simulink model "AIL_STATE_MACHINE"  (R2021b)
settings: Solver=FixedStepDiscrete  StartTime=0.0  StopTime=20  FixedStep=1e-3  RelTol=1e-3
undefined symbols (not defined in the file): BUCU3_FCC1_LHACTCMDVSCURRENTVALID, BUCU3_FCC1_LHACTCTLVSMONLOOPVALID, BUCU3_FCC1_LHACTPOSVSCMDVALID, BUCU3_FCC1_LHELEVPOSITIONVALID, BUCU3_FCC1_LHGEARINGVALID, BUCU3_FCC1_LHHYDPRESSVALID, BUCU3_FCC1_LHPOWERVALID, BUCU3_FCC1_LHSPEEDINPUTVALID, sigbuilder_block
libraries: simulink x5, LATCH_ERROR_LIB x1
settings Model: Creator=C83127  LastModifiedBy=ACH

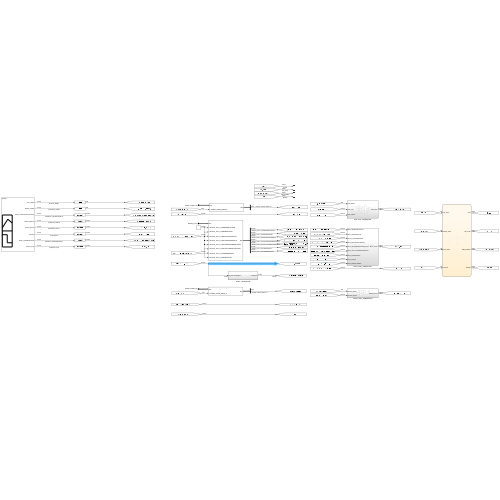
[thumbnail: Simulink's stored preview of the top-level diagram]
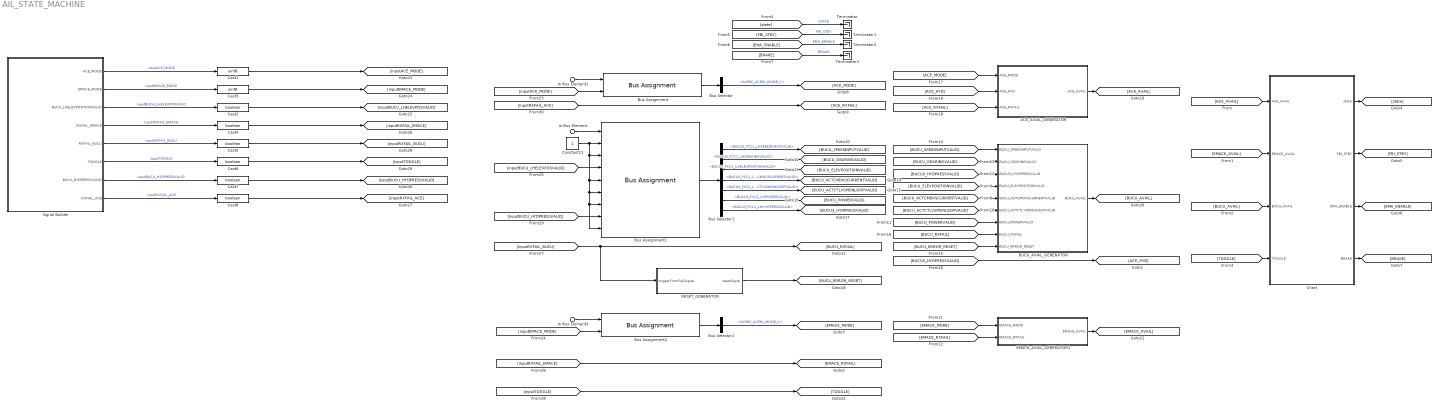
== system AIL_STATE_MACHINE ==
  In Bus Element : Inport  PortName=BUCU3_FCC1
  In Bus Element1 : Inport  Port=2  PortName=ACE9C_ACE8x_9C
  In Bus Element3 : Inport  Port=3  PortName=ACE8C_ACE9x_8C
  ACE_AVAIL_GENERATOR : Subsystem
  BUCU_AVAIL_GENERATOR : Subsystem
  Bus Assignment : BusAssignment  AssignedSignals=ACE9C_ACE8x_MODE_C
  Bus Assignment1 : BusAssignment  AssignedSignals=BUCU3_FCC1_LHSPEEDINPUTVALID,BUCU3_FCC1_LHGEARINGVALID,BUCU3_FCC1_LHELEVPOSITIONVALID,BUCU3_FCC1_LHACTPOSVSCMDVALID,BUCU3_FCC1_LHACTCMDVSCURRENTVALID,BUCU3_FCC1_LHACTCTLVSMONLOOPVALID,BUCU3_FCC1_LHHYDPRESSVALID,BUCU3_FCC1_LHPOWERVALID
  Bus Assignment2 : BusAssignment  AssignedSignals=ACE8C_ACE9x_MODE_C
  Bus Selector : BusSelector  OutputSignals=ACE9C_ACE8x_MODE_C
  Bus Selector1 : BusSelector  OutputSignals=BUCU3_FCC1_LHSPEEDINPUTVALID,BUCU3_FCC1_LHGEARINGVALID,BUCU3_FCC1_LHELEVPOSITIONVALID,BUCU3_FCC1_LHACTCMDVSCURRENTVALID,BUCU3_FCC1_LHACTCTLVSMONLOOPVALID,BUCU3_FCC1_LHPOWERVALID,BUCU3_FCC1_LHHYDPRESSVALID
  Bus Selector2 : BusSelector  OutputSignals=ACE8C_ACE9x_MODE_C
  Cast1 : DataTypeConversion  OutDataTypeStr=uint8
  Cast{2,4..8} (6 alike) : DataTypeConversion  OutDataTypeStr=boolean
  Cast3 : DataTypeConversion  OutDataTypeStr=uint8
  Chart : Stateflow chart  TreatAsAtomicUnit=on
  Constant13 : Constant  OutDataTypeStr=boolean
  EMACE_AVAIL_GENERATOR1 : Subsystem
  RESET_GENERATOR : Subsystem
  Signal Builder : Subsystem  Tag=STV Subsys  LoadFcn=sigbuilder_block('load');  StartFcn=sigbuilder_block('start');  StopFcn=sigbuilder_block('stop');  ClipboardFcn=sigbuilder_block('clipboard');  mask(Sigbuilder block){tuvar=[0:10]}
      mask help: Simulink:masks:SigbuilderBlock_MD
      mask init:
      | if ~strcmp(get_param(bdroot(gcbh),'SimulationStatus'),'stopped') tuvar = sigbuilder_block('maskInit'); end
      settings: CopyFcn=sigbuilder_block('copy');  DeleteFcn=sigbuilder_block('delete');  ModelCloseFcn=sigbuilder_block('modelClose');  PreSaveFcn=sigbuilder_block('preSave');  PauseFcn=sigbuilder_block('pause');  ContinueFcn=sigbuilder_block('continue');  NameChangeFcn=sigbuilder_block('namechange');  OpenFcn=sigbuilder_block('open',[6 30 1428 681.75 ]);  CloseFcn=sigbuilder_block('close');
      mask Display: plot(0, 0, 100, 100,[2, 2, 32, 32, 2], [68, 8, 8, 68, 68],[32, 2], [38, 38], [32, 19, 2],[53, 60, 44], [32, 17, 17, 2],[16, 16, 31, 31]);txt = getActiveGroup(gcbh);text(2, 100, txt,'verticalAlignment', 'top');
  Terminator{,1..3} (4 alike) : Terminator
  wires:
  [ACE_AVAIL] -> Chart/1(ACE_AVAIL)
  [EMACE_AVAIL] -> Chart/2(EMACE_AVAIL)
  [BUCU_AVAIL] -> Chart/3(BUCU_AVAIL)
  [TOGGLE] -> Chart/4(TOGGLE)
  Chart/1(state) -> [state]
  Chart/2(FBI_STBY) -> [FBI_STBY]
  Chart/3(EMA_ENABLE) -> [EMA_ENABLE]
  Chart/4(BRAKE) -> [BRAKE]
  [EMA_ENABLE] -> Terminator2/1  "EMA_ENABLE"
  [FBI_STBY] -> Terminator1/1  "FBI_STBY"
  [state] -> Terminator/1  "STATE"
  [BRAKE] -> Terminator3/1  "BRAKE"
  Bus Selector/1 -> [ACE_MODE]  "<ACE9C_ACE8x_MODE_C>"
  [inputRXFAIL_ACE] -> [ACE_RXFAIL]
  Bus Selector1/1 -> [BUCU_SPEEDINPUTVALID]  "<BUCU3_FCC1_LHSPEEDINPUTVALID>"
  Bus Selector1/2 -> [BUCU_GEARINGVALID]  "<BUCU3_FCC1_LHGEARINGVALID>"
  Bus Selector1/3 -> [BUCU_ELEVPOSITIONVALID]  "<BUCU3_FCC1_LHELEVPOSITIONVALID>"
  Bus Selector1/4 -> [BUCU_ACTCMDVSCURRENTVALID]  "<BUCU3_FCC1_LHACTCMDVSCURRENTVALID>"
  Bus Selector1/5 -> [BUCU_ACTCTLVSMONLOOPVALID]  "<BUCU3_FCC1_LHACTCTLVSMONLOOPVALID>"
  Bus Selector1/6 -> [BUCU_POWERVALID]  "<BUCU3_FCC1_LHPOWERVALID>"
  Bus Selector1/7 -> [BUCU3_HYDPRESSVALID]  "<BUCU3_FCC1_LHHYDPRESSVALID>"
  [BUCU_SPEEDINPUTVALID] -> BUCU_AVAIL_GENERATOR/1(BUCU_SPEEDINPUTVALID)
  [BUCU_GEARINGVALID] -> BUCU_AVAIL_GENERATOR/2(BUCU_GEARINGVALID)
  [BUCU3_HYDPRESSVALID] -> BUCU_AVAIL_GENERATOR/3(BUCU3_HYDPRESSVALID)
  [BUCU_ELEVPOSITIONVALID] -> BUCU_AVAIL_GENERATOR/4(BUCU_ELEVPOSITIONVALID)
  [BUCU_ACTCMDVSCURRENTVALID] -> BUCU_AVAIL_GENERATOR/5(BUCU_ACTCMDVSCURRENTVALID)
  [BUCU_ACTCTLVSMONLOOPVALID] -> BUCU_AVAIL_GENERATOR/6(BUCU_ACTCTLVSMONLOOPVALID)
  [BUCU_POWERVALID] -> BUCU_AVAIL_GENERATOR/7(BUCU_POWERVALID)
  [BUCU_ERROR_RESET] -> BUCU_AVAIL_GENERATOR/9(BUCU_ERROR_RESET)
  BUCU_AVAIL_GENERATOR/1(BUCU_AVAIL) -> [BUCU_AVAIL]
  [BUCU_RXFAIL] -> BUCU_AVAIL_GENERATOR/8(BUCU_RXFAIL)
  In Bus Element1/1 -> Bus Assignment/1
  In Bus Element/1 -> Bus Assignment1/1
  [inputRXFAIL_BUCU] -> RESET_GENERATOR/1(triggerFromFailSignal), [BUCU_RXFAIL]
  [ACE_MODE] -> ACE_AVAIL_GENERATOR/1(ACE_MODE)
  [ACE_HYD] -> ACE_AVAIL_GENERATOR/2(ACE_HYD)
  [ACE_RXFAIL] -> ACE_AVAIL_GENERATOR/3(ACE_RXFAIL)
  ACE_AVAIL_GENERATOR/1(ACE_AVAIL) -> [ACE_AVAIL]
  [BUCU3_HYDPRESSVALID] -> [ACE_HYD]
  In Bus Element3/1 -> Bus Assignment2/1
  [inputRXFAIL_EMACE] -> [EMACE_RXFAIL]
  Bus Selector2/1 -> [EMACE_MODE]  "<ACE8C_ACE9x_MODE_C>"
  [EMACE_RXFAIL] -> EMACE_AVAIL_GENERATOR1/2(EMACE_RXFAIL)
  [EMACE_MODE] -> EMACE_AVAIL_GENERATOR1/1(EMACE_MODE)
  EMACE_AVAIL_GENERATOR1/1(EMACE_AVAIL) -> [EMACE_AVAIL]
  Bus Assignment/1 -> Bus Selector/1
  [inputACE_MODE] -> Bus Assignment/2
  Bus Assignment1/1 -> Bus Selector1/1
  Constant13/1 -> Bus Assignment1/5, Bus Assignment1/6, Bus Assignment1/7, Bus Assignment1/9, Bus Assignment1/3, Bus Assignment1/2
  [inputBUCU_HYDPRESSVALID] -> Bus Assignment1/8
  Bus Assignment2/1 -> Bus Selector2/1
  [inputEMACE_MODE] -> Bus Assignment2/2
  [inputTOGGLE] -> [TOGGLE]
  Signal Builder/1(ACE_MODE) -> Cast1/1  "inputACE_MODE"
  Signal Builder/2(EMACE_MODE) -> Cast3/1  "inputEMACE_MODE"
  Signal Builder/3(BUCU_LHELEVPOSITIONVALID) -> Cast2/1  "inputBUCU_LHELEVPOSVALID"
  Signal Builder/4(RXFAIL_EMACE) -> Cast4/1  "inputRXFAIL_EMACE"
  Signal Builder/8(RXFAIL_ACE) -> Cast8/1  "inputRXFAIL_ACE"
  Signal Builder/5(RXFAIL_BUCU) -> Cast5/1  "inputRXFAIL_BUCU"
  Signal Builder/6(TOGGLE) -> Cast6/1  "inputTOGGLE"
  Signal Builder/7(BUCU_HYDPRESSVALID) -> Cast7/1  "inputBUCU_HYDPRESSVALID"
  [inputBUCU_LHELEVPOSVALID] -> Bus Assignment1/4
  Cast1/1 -> [inputACE_MODE]
  Cast3/1 -> [inputEMACE_MODE]
  Cast2/1 -> [inputBUCU_LHELEVPOSVALID]
  Cast4/1 -> [inputRXFAIL_EMACE]
  Cast5/1 -> [inputRXFAIL_BUCU]
  Cast6/1 -> [inputTOGGLE]
  Cast7/1 -> [inputBUCU_HYDPRESSVALID]
  Cast8/1 -> [inputRXFAIL_ACE]
  RESET_GENERATOR/1(resetSignal) -> [BUCU_ERROR_RESET]

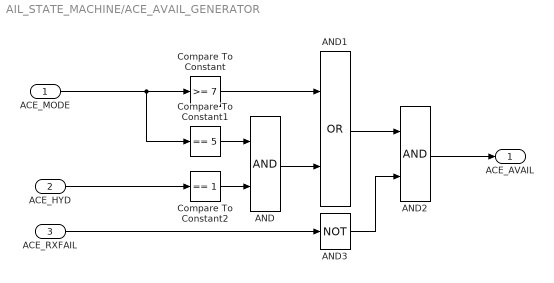
== system AIL_STATE_MACHINE/ACE_AVAIL_GENERATOR ==
  ACE_MODE : Inport
  ACE_HYD : Inport  Port=2
  ACE_RXFAIL : Inport  Port=3
  AND : Logic  AllPortsSameDT=off  OutDataTypeStr=boolean
  AND1 : Logic  Operator=OR  AllPortsSameDT=off  OutDataTypeStr=boolean
  AND2 : Logic  AllPortsSameDT=off  OutDataTypeStr=boolean
  AND3 : Logic  Operator=NOT  AllPortsSameDT=off  OutDataTypeStr=boolean
  Compare To Constant : simulink/Logic and Bit Operations/Compare To Constant  relop=>=  const=7  OutDataTypeStr=boolean
  Compare To Constant1 : simulink/Logic and Bit Operations/Compare To Constant  relop===  const=5  OutDataTypeStr=boolean
  Compare To Constant2 : simulink/Logic and Bit Operations/Compare To Constant  relop===  const=1  OutDataTypeStr=boolean
  ACE_AVAIL : Outport
  wires:
  AND3/1 -> AND2/2
  AND/1 -> AND1/2
  AND1/1 -> AND2/1
  Compare To Constant1/1 -> AND/1
  Compare To Constant2/1 -> AND/2
  ACE_MODE/1 -> Compare To Constant1/1, Compare To Constant/1
  Compare To Constant/1 -> AND1/1
  AND2/1 -> ACE_AVAIL/1
  ACE_HYD/1 -> Compare To Constant2/1
  ACE_RXFAIL/1 -> AND3/1

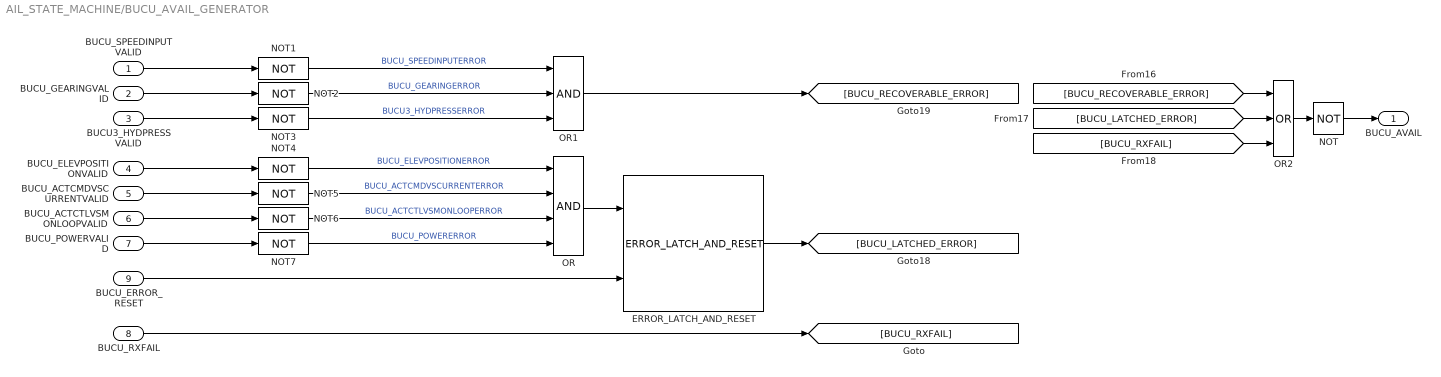
== system AIL_STATE_MACHINE/BUCU_AVAIL_GENERATOR ==
  BUCU_SPEEDINPUTVALID : Inport
  BUCU_GEARINGVALID : Inport  Port=2
  BUCU3_HYDPRESSVALID : Inport  Port=3
  BUCU_ELEVPOSITIONVALID : Inport  Port=4
  BUCU_ACTCMDVSCURRENTVALID : Inport  Port=5
  BUCU_ACTCTLVSMONLOOPVALID : Inport  Port=6
  BUCU_POWERVALID : Inport  Port=7
  BUCU_RXFAIL : Inport  Port=8
  BUCU_ERROR_RESET : Inport  Port=9
  ERROR_LATCH_AND_RESET : LATCH_ERROR_LIB/ERROR_LATCH_AND_RESET  SystemSampleTime=-1  VariantActivationTime=update diagram  Latency=0  AutoFrameSizeCalculation=off
  NOT : Logic  Operator=NOT  IconShape=distinctive  AllPortsSameDT=off  OutDataTypeStr=boolean
  NOT{1..7} (7 alike) : Logic  Operator=NOT  AllPortsSameDT=off  OutDataTypeStr=boolean
  OR : Logic  Inputs=4  AllPortsSameDT=off  OutDataTypeStr=boolean
  OR1 : Logic  Inputs=3  AllPortsSameDT=off  OutDataTypeStr=boolean
  OR2 : Logic  Operator=OR  Inputs=3  AllPortsSameDT=off  OutDataTypeStr=boolean
  BUCU_AVAIL : Outport
  wires:
  ERROR_LATCH_AND_RESET/1 -> [BUCU_LATCHED_ERROR]
  OR2/1 -> NOT/1
  NOT/1 -> BUCU_AVAIL/1
  [BUCU_RECOVERABLE_ERROR] -> OR2/1
  OR/1 -> ERROR_LATCH_AND_RESET/1
  OR1/1 -> [BUCU_RECOVERABLE_ERROR]
  BUCU_ACTCMDVSCURRENTVALID/1 -> NOT5/1
  [BUCU_RXFAIL] -> OR2/3
  [BUCU_LATCHED_ERROR] -> OR2/2
  BUCU_ELEVPOSITIONVALID/1 -> NOT4/1
  BUCU_POWERVALID/1 -> NOT7/1
  BUCU3_HYDPRESSVALID/1 -> NOT3/1
  BUCU_ACTCTLVSMONLOOPVALID/1 -> NOT6/1
  BUCU_ERROR_RESET/1 -> ERROR_LATCH_AND_RESET/2
  BUCU_GEARINGVALID/1 -> NOT2/1
  BUCU_SPEEDINPUTVALID/1 -> NOT1/1
  BUCU_RXFAIL/1 -> [BUCU_RXFAIL]
  NOT1/1 -> OR1/1  "BUCU_SPEEDINPUTERROR"
  NOT2/1 -> OR1/2  "BUCU_GEARINGERROR"
  NOT3/1 -> OR1/3  "BUCU3_HYDPRESSERROR"
  NOT4/1 -> OR/1  "BUCU_ELEVPOSITIONERROR"
  NOT5/1 -> OR/2  "BUCU_ACTCMDVSCURRENTERROR"
  NOT6/1 -> OR/3  "BUCU_ACTCTLVSMONLOOPERROR"
  NOT7/1 -> OR/4  "BUCU_POWERERROR"

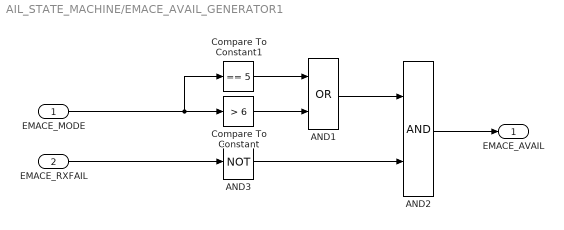
== system AIL_STATE_MACHINE/EMACE_AVAIL_GENERATOR1 ==
  EMACE_MODE : Inport
  EMACE_RXFAIL : Inport  Port=2
  AND1 : Logic  Operator=OR  AllPortsSameDT=off  OutDataTypeStr=boolean
  AND2 : Logic  AllPortsSameDT=off  OutDataTypeStr=boolean
  AND3 : Logic  Operator=NOT  AllPortsSameDT=off  OutDataTypeStr=boolean
  Compare To Constant : simulink/Logic and Bit Operations/Compare To Constant  relop=>  const=6  OutDataTypeStr=boolean
  Compare To Constant1 : simulink/Logic and Bit Operations/Compare To Constant  relop===  const=5  OutDataTypeStr=boolean
  EMACE_AVAIL : Outport
  wires:
  EMACE_RXFAIL/1 -> AND3/1
  AND2/1 -> EMACE_AVAIL/1
  EMACE_MODE/1 -> Compare To Constant1/1, Compare To Constant/1
  Compare To Constant/1 -> AND1/2
  AND3/1 -> AND2/2
  AND1/1 -> AND2/1
  Compare To Constant1/1 -> AND1/1

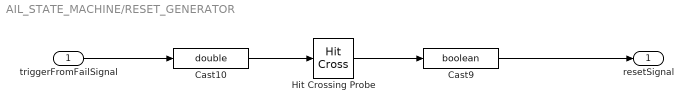
== system AIL_STATE_MACHINE/RESET_GENERATOR ==
  triggerFromFailSignal : Inport
  Cast10 : DataTypeConversion  OutDataTypeStr=double
  Cast9 : DataTypeConversion  OutDataTypeStr=boolean
  Hit Crossing Probe : HitCross  HitCrossingOffset=0.5  HitCrossingDirection=falling
  resetSignal : Outport
  wires:
  Cast10/1 -> Hit Crossing Probe/1
  Hit Crossing Probe/1 -> Cast9/1
  triggerFromFailSignal/1 -> Cast10/1
  Cast9/1 -> resetSignal/1

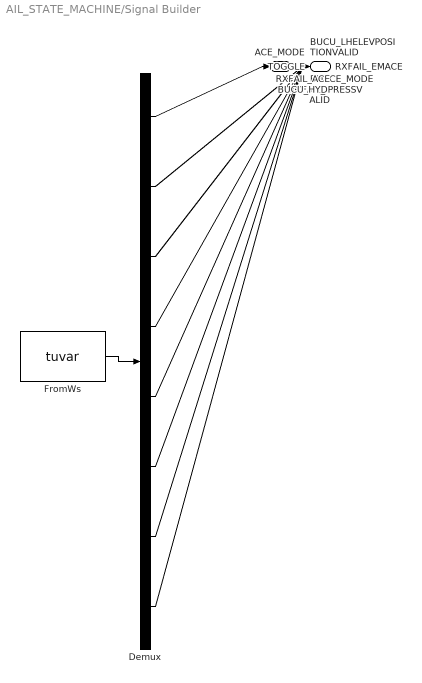
== system AIL_STATE_MACHINE/Signal Builder ==
  Demux : Demux  Tag=STV Demux  Outputs=8
      settings: DisplayOption=none
  FromWs : FromWorkspace  Tag=STV FromWs  VariableName=tuvar
      SigBuilderData=|
      | common.afterFinalStr = 'Extrapolate'
      | common.sampleTime = 0
      | dataSet.timeRange = [0 20]
      | dataSet.name = 'Group 1'
      | sbobj.Groups.Name = 'Group 1'
      | sbobj.Groups.Signals(1).Name = 'ACE_MODE'
      | sbobj.Groups.Signals(1).XData = [0 1.5 1.5 18 18 20]
      | sbobj.Groups.Signals(1).YData = [1 1 7 7 1 1]
      | sbobj.Groups.Signals(2).Name = 'EMACE_MODE'
      | sbobj.Groups.Signals(2).XData = [0 2 2 18 18 20]
      | sbobj.Groups.Signals(2).YData = [1 1 7 7 1 1]
      | sbobj.Groups.Signals(3).Name = 'BUCU_LHELEVPOSITIONVALID'
      | sbobj.Groups.Signals(3).XData = [0 1 13 13 14 14 20]
      | sbobj.Groups.Signals(3).YData = [1 1 1 0 0 1 1]
      | sbobj.Groups.Signals(4).Name = 'RXFAIL_EMACE'
      | sbobj.Groups.Signals(4).XData = [0 3 3 4 4 7 7 7.5 7.5 20]
      | sbobj.Groups.Signals(4).YData = [0 0 1 1 0 0 1 1 0 0]
      | sbobj.Groups.Signals(5).Name = 'RXFAIL_BUCU'
      | sbobj.Groups.Signals(5).XData = [0 3.5 3.5 5 5 20]
      | sbobj.Groups.Signals(5).YData = [0 0 1 1 0 0]
      | sbobj.Groups.Signals(6).Name = 'TOGGLE'
      | sbobj.Groups.Signals(6).XData = [0 6 6 8 8 10 10 12 12 20]
      | sbobj.Groups.Signals(6).YData = [0 0 1 1 0 0 1 1 0 0]
      | sbobj.Groups.Signals(7).Name = 'BUCU_HYDPRESSVALID'
      | sbobj.Groups.Signals(7).XData = [0 8.5 8.5 9.5 9.5 20]
      | sbobj.Groups.Signals(7).YData = [1 1 0 0 1 1]
      | sbobj.Groups.Signals(8).Name = 'RXFAIL_ACE'
      | sbobj.Groups.Signals(8).XData = [0 2.5 2.5 4.5 4.5 20]
      | sbobj.Groups.Signals(8).YData = [0 0 1 1 0 0]
      | sbobj.Groups.TimeRange = [0 20]
  ACE_MODE : Outport  Tag=STV Outport
  EMACE_MODE : Outport  Tag=STV Outport  Port=2
  BUCU_LHELEVPOSITIONVALID : Outport  Tag=STV Outport  Port=3
  RXFAIL_EMACE : Outport  Tag=STV Outport  Port=4
  RXFAIL_BUCU : Outport  Tag=STV Outport  Port=5
  TOGGLE : Outport  Tag=STV Outport  Port=6
  BUCU_HYDPRESSVALID : Outport  Tag=STV Outport  Port=7
  RXFAIL_ACE : Outport  Tag=STV Outport  Port=8
  wires:
  FromWs/1 -> Demux/1
  Demux/1 -> ACE_MODE/1
  Demux/2 -> EMACE_MODE/1
  Demux/3 -> BUCU_LHELEVPOSITIONVALID/1
  Demux/4 -> RXFAIL_EMACE/1
  Demux/5 -> RXFAIL_BUCU/1
  Demux/6 -> TOGGLE/1
  Demux/7 -> BUCU_HYDPRESSVALID/1
  Demux/8 -> RXFAIL_ACE/1

== stateflow chart AIL_STATE_MACHINE/Chart ==
  state LOSS
    state = 0;
    FBI_STBY = 0;
    EMA_ENABLE = 0;
    BRAKE = 1;
  state HYDRAULIC
    state = 1;
    FBI_STBY = 0;
    EMA_ENABLE = 0;
    BRAKE = 0;
  state ELECTRIC
    state = 2;
    FBI_STBY = 1;
    EMA_ENABLE = 1;
    BRAKE = 0;
  state BACKUP
    state = 3;
    FBI_STBY = 0;
    EMA_ENABLE = 0;
    BRAKE = 0;
  (default) -> LOSS
  ELECTRIC -> LOSS : [(EMACE_AVAIL == 0) | ...
      | ((ACE_AVAIL == 1) & (TOGGLE == 0))]
  HYDRAULIC -> LOSS : [(ACE_AVAIL == 0) | ...
      | ((ACE_AVAIL== 1) & (TOGGLE == 1) & (EMACE_AVAIL == 1))]
  LOSS -> ELECTRIC [order 2] : [((EMACE_AVAIL == 1) & (TOGGLE == 1)) | ...
      | ((EMACE_AVAIL == 1) & (ACE_AVAIL == 0))]
  LOSS -> HYDRAULIC [order 1] : [((ACE_AVAIL == 1) & (TOGGLE == 0)) | ...
      | (EMACE_AVAIL == 0) & (ACE_AVAIL == 1)]
  LOSS -> BACKUP [order 3] : [(ACE_AVAIL == 0) & (EMACE_AVAIL == 0) & (BUCU_AVAIL == 1)]
  BACKUP -> LOSS : [(BUCU_AVAIL == 0) | ...
      | ((ACE_AVAIL == 1) | (EMACE_AVAIL == 1))]
  data: ACE_AVAIL input; EMACE_AVAIL input; BUCU_AVAIL input; TOGGLE input; state output; FBI_STBY output; EMA_ENABLE output; BRAKE output
